simulink model "Blocks"  (R2020a)
settings: Solver=VariableStepAuto  StartTime=0.0  StopTime=10.0  RelTol=1e-3
libraries: simulink x3
settings Model: Creator=kohmeikadoya  LastModifiedBy=kohmeikadoya

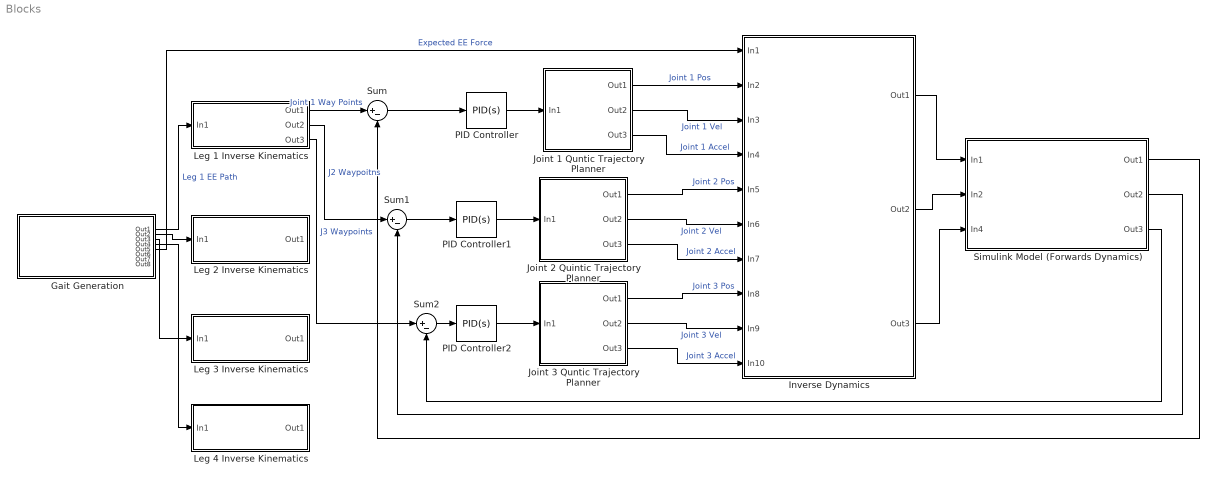
== system Blocks ==
  Gait Generation : Subsystem
      mask Display: image('/Users/kohmeikadoya/Desktop/Screen Shot 2021-05-12 at 1.38.06 AM.png'); % Use "Edit Image" on toolstrip to change.
  Inverse Dynamics : Subsystem
      mask Display: image('/Users/kohmeikadoya/Desktop/Screen Shot 2021-05-12 at 1.58.14 AM.png'); % Use "Edit Image" on toolstrip to change.
  Joint 1 Quntic Trajectory Planner : Subsystem
      mask Display: image('/Users/kohmeikadoya/Desktop/Screen Shot 2021-05-12 at 1.48.20 AM.png'); % Use "Edit Image" on toolstrip to change.
  Joint 2 Quintic Trajectory Planner : Subsystem
      mask Display: image('/Users/kohmeikadoya/Desktop/Screen Shot 2021-05-12 at 1.48.20 AM.png'); % Use "Edit Image" on toolstrip to change.
  Joint 3 Quntic Trajectory Planner : Subsystem
      mask Display: image('/Users/kohmeikadoya/Desktop/Screen Shot 2021-05-12 at 1.48.20 AM.png'); % Use "Edit Image" on toolstrip to change.
  Leg 1 Inverse Kinematics : Subsystem
      mask Display: image('/Users/kohmeikadoya/Downloads/InvKine.png'); % Use "Edit Image" on toolstrip to change.
  Leg 2 Inverse Kinematics : Subsystem
      mask Display: image('/Users/kohmeikadoya/Downloads/InvKine.png'); % Use "Edit Image" on toolstrip to change.
  Leg 3 Inverse Kinematics : Subsystem
      mask Display: image('/Users/kohmeikadoya/Downloads/InvKine.png'); % Use "Edit Image" on toolstrip to change.
  Leg 4 Inverse Kinematics : Subsystem
      mask Display: image('/Users/kohmeikadoya/Downloads/InvKine.png'); % Use "Edit Image" on toolstrip to change.
  PID Controller : simulink/Continuous/PID Controller  Controller=PID  Form=Parallel  TimeDomain=Continuous-time  UseExternalTs=off  SampleTime=-1  IntegratorMethod=Forward Euler  FilterMethod=Forward Euler  ControllerParametersSource=internal  P=1  I=1  D=0  UseFilter=on  N=100  TunerSelectOption=Transfer Function Based (PID Tuner App)  InitialConditionSource=internal  InitialConditionForIntegrator=0  InitialConditionForFilter=0  DifferentiatorICPrevScaledInput=0  ExternalReset=none  TrackingMode=off  Kt=1  LimitOutput=off  UpperSaturationLimit=inf  LowerSaturationLimit=-inf  LinearizeAsGain=on  AntiWindupMode=none  Kb=1  POutMin=[]  POutMax=[]  IOutMin=[]  IOutMax=[]  DOutMin=[]  DOutMax=[]  NOutMin=[]  NOutMax=[]  SumOutMin=[]  SumOutMax=[]  SaturationOutMin=[]  SaturationOutMax=[]  PParamMin=[]  PParamMax=[]  IParamMin=[]  IParamMax=[]  DParamMin=[]  DParamMax=[]  NParamMin=[]  NParamMax=[]  KbParamMin=[]  KbParamMax=[]  KtParamMin=[]  KtParamMax=[]  KbOutMin=[]  KbOutMax=[]  KtOutMin=[]  KtOutMax=[]  IntegratorOutMin=[]  IntegratorOutMax=[]  FilterOutMin=[]  FilterOutMax=[]  SumI1OutMin=[]  SumI1OutMax=[]  SumI2OutMin=[]  SumI2OutMax=[]  SumI3OutMin=[]  SumI3OutMax=[]  SumI4OutMin=[]  SumI4OutMax=[]  SumDOutMin=[]  SumDOutMax=[]  DifferentiatorOutMin=[]  DifferentiatorOutMax=[]  FilterDiffOutCoefMin=[]  FilterDiffOutCoefMax=[]  ReciprocalOutMin=[]  ReciprocalOutMax=[]  SumDenOutMin=[]  SumDenOutMax=[]  SumNumOutMin=[]  SumNumOutMax=[]  DivideOutMin=[]  DivideOutMax=[]  UdiffTsProdOutMin=[]  UdiffTsProdOutMax=[]  NTsProdOutMin=[]  NTsProdOutMax=[]  UintegralTsProdOutMin=[]  UintegralTsProdOutMax=[]  UngainTsProdOutMin=[]  UngainTsProdOutMax=[]  IntegratorContinuousStateAttributes=''  IntegratorStateMustResolveToSignalObject=off  IntegratorRTWStateStorageClass=Auto  FilterContinuousStateAttributes=''  FilterStateMustResolveToSignalObject=off  FilterRTWStateStorageClass=Auto  ParallelPVariant=InternalParameters  IdealPVariant=Disabled  IVariant=InternalParameters  DVariant=InternalParameters  IntegratorVariant=Continuous  SatVariant=Disabled  AWVariant=Passthrough  PCopyVariant=Disabled  TRVariant=Disabled  FdbkBlocksVariant=Forward  IdealPFdbkVariant=Disabled  SatFdbkVariant=Disabled  DerivativeFilterVariant=ContFilter  NVariant=InternalParameters  NCopyVariant=Disabled  FilterICVariant=InternalICsFilter  IntegratorICVariant=InternalICs  ExternalResetVariant=Disabled  TRSumVariant=Passthrough  SumFdbkVariant=Disabled  SumVariant=Sum_PID  TsampFilterVariant=InternalTs  TsampNgainVariant=Passthrough  TsampIntegralVariant=Passthrough
  PID Controller1 : simulink/Continuous/PID Controller  Controller=PID  Form=Parallel  TimeDomain=Continuous-time  UseExternalTs=off  SampleTime=-1  IntegratorMethod=Forward Euler  FilterMethod=Forward Euler  ControllerParametersSource=internal  P=1  I=1  D=0  UseFilter=on  N=100  TunerSelectOption=Transfer Function Based (PID Tuner App)  InitialConditionSource=internal  InitialConditionForIntegrator=0  InitialConditionForFilter=0  DifferentiatorICPrevScaledInput=0  ExternalReset=none  TrackingMode=off  Kt=1  LimitOutput=off  UpperSaturationLimit=inf  LowerSaturationLimit=-inf  LinearizeAsGain=on  AntiWindupMode=none  Kb=1  POutMin=[]  POutMax=[]  IOutMin=[]  IOutMax=[]  DOutMin=[]  DOutMax=[]  NOutMin=[]  NOutMax=[]  SumOutMin=[]  SumOutMax=[]  SaturationOutMin=[]  SaturationOutMax=[]  PParamMin=[]  PParamMax=[]  IParamMin=[]  IParamMax=[]  DParamMin=[]  DParamMax=[]  NParamMin=[]  NParamMax=[]  KbParamMin=[]  KbParamMax=[]  KtParamMin=[]  KtParamMax=[]  KbOutMin=[]  KbOutMax=[]  KtOutMin=[]  KtOutMax=[]  IntegratorOutMin=[]  IntegratorOutMax=[]  FilterOutMin=[]  FilterOutMax=[]  SumI1OutMin=[]  SumI1OutMax=[]  SumI2OutMin=[]  SumI2OutMax=[]  SumI3OutMin=[]  SumI3OutMax=[]  SumI4OutMin=[]  SumI4OutMax=[]  SumDOutMin=[]  SumDOutMax=[]  DifferentiatorOutMin=[]  DifferentiatorOutMax=[]  FilterDiffOutCoefMin=[]  FilterDiffOutCoefMax=[]  ReciprocalOutMin=[]  ReciprocalOutMax=[]  SumDenOutMin=[]  SumDenOutMax=[]  SumNumOutMin=[]  SumNumOutMax=[]  DivideOutMin=[]  DivideOutMax=[]  UdiffTsProdOutMin=[]  UdiffTsProdOutMax=[]  NTsProdOutMin=[]  NTsProdOutMax=[]  UintegralTsProdOutMin=[]  UintegralTsProdOutMax=[]  UngainTsProdOutMin=[]  UngainTsProdOutMax=[]  IntegratorContinuousStateAttributes=''  IntegratorStateMustResolveToSignalObject=off  IntegratorRTWStateStorageClass=Auto  FilterContinuousStateAttributes=''  FilterStateMustResolveToSignalObject=off  FilterRTWStateStorageClass=Auto  ParallelPVariant=InternalParameters  IdealPVariant=Disabled  IVariant=InternalParameters  DVariant=InternalParameters  IntegratorVariant=Continuous  SatVariant=Disabled  AWVariant=Passthrough  PCopyVariant=Disabled  TRVariant=Disabled  FdbkBlocksVariant=Forward  IdealPFdbkVariant=Disabled  SatFdbkVariant=Disabled  DerivativeFilterVariant=ContFilter  NVariant=InternalParameters  NCopyVariant=Disabled  FilterICVariant=InternalICsFilter  IntegratorICVariant=InternalICs  ExternalResetVariant=Disabled  TRSumVariant=Passthrough  SumFdbkVariant=Disabled  SumVariant=Sum_PID  TsampFilterVariant=InternalTs  TsampNgainVariant=Passthrough  TsampIntegralVariant=Passthrough
  PID Controller2 : simulink/Continuous/PID Controller  Controller=PID  Form=Parallel  TimeDomain=Continuous-time  UseExternalTs=off  SampleTime=-1  IntegratorMethod=Forward Euler  FilterMethod=Forward Euler  ControllerParametersSource=internal  P=1  I=1  D=0  UseFilter=on  N=100  TunerSelectOption=Transfer Function Based (PID Tuner App)  InitialConditionSource=internal  InitialConditionForIntegrator=0  InitialConditionForFilter=0  DifferentiatorICPrevScaledInput=0  ExternalReset=none  TrackingMode=off  Kt=1  LimitOutput=off  UpperSaturationLimit=inf  LowerSaturationLimit=-inf  LinearizeAsGain=on  AntiWindupMode=none  Kb=1  POutMin=[]  POutMax=[]  IOutMin=[]  IOutMax=[]  DOutMin=[]  DOutMax=[]  NOutMin=[]  NOutMax=[]  SumOutMin=[]  SumOutMax=[]  SaturationOutMin=[]  SaturationOutMax=[]  PParamMin=[]  PParamMax=[]  IParamMin=[]  IParamMax=[]  DParamMin=[]  DParamMax=[]  NParamMin=[]  NParamMax=[]  KbParamMin=[]  KbParamMax=[]  KtParamMin=[]  KtParamMax=[]  KbOutMin=[]  KbOutMax=[]  KtOutMin=[]  KtOutMax=[]  IntegratorOutMin=[]  IntegratorOutMax=[]  FilterOutMin=[]  FilterOutMax=[]  SumI1OutMin=[]  SumI1OutMax=[]  SumI2OutMin=[]  SumI2OutMax=[]  SumI3OutMin=[]  SumI3OutMax=[]  SumI4OutMin=[]  SumI4OutMax=[]  SumDOutMin=[]  SumDOutMax=[]  DifferentiatorOutMin=[]  DifferentiatorOutMax=[]  FilterDiffOutCoefMin=[]  FilterDiffOutCoefMax=[]  ReciprocalOutMin=[]  ReciprocalOutMax=[]  SumDenOutMin=[]  SumDenOutMax=[]  SumNumOutMin=[]  SumNumOutMax=[]  DivideOutMin=[]  DivideOutMax=[]  UdiffTsProdOutMin=[]  UdiffTsProdOutMax=[]  NTsProdOutMin=[]  NTsProdOutMax=[]  UintegralTsProdOutMin=[]  UintegralTsProdOutMax=[]  UngainTsProdOutMin=[]  UngainTsProdOutMax=[]  IntegratorContinuousStateAttributes=''  IntegratorStateMustResolveToSignalObject=off  IntegratorRTWStateStorageClass=Auto  FilterContinuousStateAttributes=''  FilterStateMustResolveToSignalObject=off  FilterRTWStateStorageClass=Auto  ParallelPVariant=InternalParameters  IdealPVariant=Disabled  IVariant=InternalParameters  DVariant=InternalParameters  IntegratorVariant=Continuous  SatVariant=Disabled  AWVariant=Passthrough  PCopyVariant=Disabled  TRVariant=Disabled  FdbkBlocksVariant=Forward  IdealPFdbkVariant=Disabled  SatFdbkVariant=Disabled  DerivativeFilterVariant=ContFilter  NVariant=InternalParameters  NCopyVariant=Disabled  FilterICVariant=InternalICsFilter  IntegratorICVariant=InternalICs  ExternalResetVariant=Disabled  TRSumVariant=Passthrough  SumFdbkVariant=Disabled  SumVariant=Sum_PID  TsampFilterVariant=InternalTs  TsampNgainVariant=Passthrough  TsampIntegralVariant=Passthrough
  Simulink Model (Forwards Dynamics) : Subsystem
      mask Display: image('/Users/kohmeikadoya/Desktop/Screen Shot 2021-05-12 at 2.00.07 AM.png'); % Use "Edit Image" on toolstrip to change.
  Sum : Sum  Inputs=|+-
  Sum1 : Sum  Inputs=|+-
  Sum2 : Sum  Inputs=|+-
  wires:
  Gait Generation/1(Out1) -> Leg 1 Inverse Kinematics/1(In1)  "Leg 1 EE Path"
  Gait Generation/2(Out2) -> Leg 2 Inverse Kinematics/1(In1)
  Gait Generation/3(Out3) -> Leg 3 Inverse Kinematics/1(In1)
  Gait Generation/4(Out4) -> Leg 4 Inverse Kinematics/1(In1)
  Gait Generation/5(Out5) -> Inverse Dynamics/1(In1)  "Expected EE Force"
  Joint 1 Quntic Trajectory Planner/1(Out1) -> Inverse Dynamics/2(In2)  "Joint 1 Pos"
  Joint 1 Quntic Trajectory Planner/2(Out2) -> Inverse Dynamics/3(In3)  "Joint 1 Vel"
  Joint 1 Quntic Trajectory Planner/3(Out3) -> Inverse Dynamics/4(In4)  "Joint 1 Accel"
  Joint 2 Quintic Trajectory Planner/1(Out1) -> Inverse Dynamics/5(In5)  "Joint 2 Pos"
  Joint 2 Quintic Trajectory Planner/2(Out2) -> Inverse Dynamics/6(In6)  "Joint 2 Vel"
  Joint 2 Quintic Trajectory Planner/3(Out3) -> Inverse Dynamics/7(In7)  "Joint 2 Accel"
  Joint 3 Quntic Trajectory Planner/1(Out1) -> Inverse Dynamics/8(In8)  "Joint 3 Pos"
  Joint 3 Quntic Trajectory Planner/2(Out2) -> Inverse Dynamics/9(In9)  "Joint 3 Vel"
  Joint 3 Quntic Trajectory Planner/3(Out3) -> Inverse Dynamics/10(In10)  "Joint 3 Accel"
  Inverse Dynamics/1(Out1) -> Simulink Model (Forwards Dynamics)/1(In1)
  Inverse Dynamics/2(Out2) -> Simulink Model (Forwards Dynamics)/2(In2)
  Inverse Dynamics/3(Out3) -> Simulink Model (Forwards Dynamics)/3(In4)
  Simulink Model (Forwards Dynamics)/1(Out1) -> Sum/2
  Leg 1 Inverse Kinematics/1(Out1) -> Sum/1  "Joint 1 Way Points"
  Sum/1 -> PID Controller/1
  PID Controller/1 -> Joint 1 Quntic Trajectory Planner/1(In1)
  Leg 1 Inverse Kinematics/2(Out2) -> Sum1/1  "J2 Waypoitns"
  Sum2/1 -> PID Controller2/1
  Sum1/1 -> PID Controller1/1
  Leg 1 Inverse Kinematics/3(Out3) -> Sum2/1  "J3 Waypoints"
  Simulink Model (Forwards Dynamics)/2(Out2) -> Sum1/2
  Simulink Model (Forwards Dynamics)/3(Out3) -> Sum2/2
  PID Controller1/1 -> Joint 2 Quintic Trajectory Planner/1(In1)
  PID Controller2/1 -> Joint 3 Quntic Trajectory Planner/1(In1)

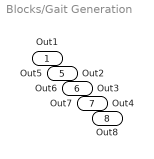
== system Blocks/Gait Generation ==
  Out1 : Outport
  Out2 : Outport  Port=2
  Out3 : Outport  Port=3
  Out4 : Outport  Port=4
  Out5 : Outport  Port=5
  Out6 : Outport  Port=6
  Out7 : Outport  Port=7
  Out8 : Outport  Port=8
  wires:
  ? -> Out1/1

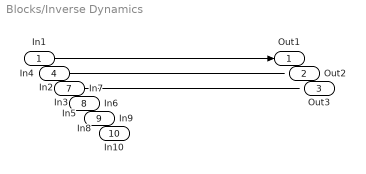
== system Blocks/Inverse Dynamics ==
  In1 : Inport
  In2 : Inport  Port=2
  In3 : Inport  Port=3
  In4 : Inport  Port=4
  In5 : Inport  Port=5
  In6 : Inport  Port=6
  In7 : Inport  Port=7
  In8 : Inport  Port=8
  In9 : Inport  Port=9
  In10 : Inport  Port=10
  Out1 : Outport
  Out2 : Outport  Port=2
  Out3 : Outport  Port=3
  wires:
  In1/1 -> Out1/1
  In4/1 -> ?
  In7/1 -> ?

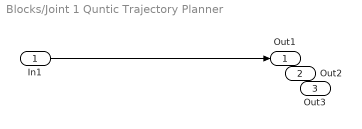
== system Blocks/Joint 1 Quntic Trajectory Planner ==
  In1 : Inport
  Out1 : Outport
  Out2 : Outport  Port=2
  Out3 : Outport  Port=3
  wires:
  In1/1 -> Out1/1

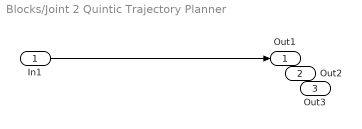
== system Blocks/Joint 2 Quintic Trajectory Planner ==
  In1 : Inport
  Out1 : Outport
  Out2 : Outport  Port=2
  Out3 : Outport  Port=3
  wires:
  In1/1 -> Out1/1

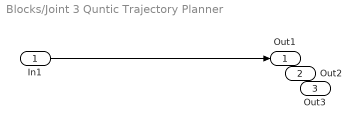
== system Blocks/Joint 3 Quntic Trajectory Planner ==
  In1 : Inport
  Out1 : Outport
  Out2 : Outport  Port=2
  Out3 : Outport  Port=3
  wires:
  In1/1 -> Out1/1

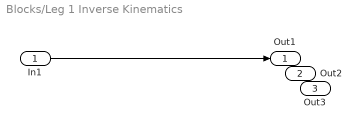
== system Blocks/Leg 1 Inverse Kinematics ==
  In1 : Inport
  Out1 : Outport
  Out2 : Outport  Port=2
  Out3 : Outport  Port=3
  wires:
  In1/1 -> Out1/1

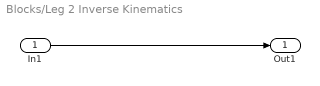
== system Blocks/Leg 2 Inverse Kinematics ==
  In1 : Inport
  Out1 : Outport
  wires:
  In1/1 -> Out1/1

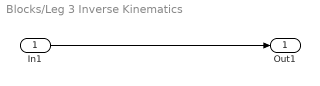
== system Blocks/Leg 3 Inverse Kinematics ==
  In1 : Inport
  Out1 : Outport
  wires:
  In1/1 -> Out1/1

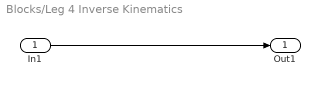
== system Blocks/Leg 4 Inverse Kinematics ==
  In1 : Inport
  Out1 : Outport
  wires:
  In1/1 -> Out1/1

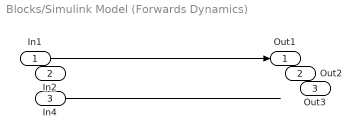
== system Blocks/Simulink Model (Forwards Dynamics) ==
  In1 : Inport
  In2 : Inport  Port=2
  In4 : Inport  Port=3
  Out1 : Outport
  Out2 : Outport  Port=2
  Out3 : Outport  Port=3
  wires:
  In1/1 -> Out1/1
  In4/1 -> ?
  ? -> ?
